simulink model "exercise2_1"  (R2025a)
settings: Solver=FixedStepAuto  StartTime=0.0  StopTime=20  FixedStep=1e-5  RelTol=1e-3
values from neighbouring files (symbols this model uses):
  B = 0    [exercise2_1.m]
  J = 2.52e-3    (= 0.00252)    [exercise2_1.m]
  K = 0.4078    [exercise2_1.m]
  Ki = 0.8    [exercise2_1.m]
  Kp = 0.1    [exercise2_1.m]
  L = 1.7e-3    (= 0.0017)    [exercise2_1.m]
  R = 0.26    [exercise2_1.m]
  wn = 2*pi*350    (= 2199.11485751)    [exercise2_1.m]
  Ww = 60    [exercise2_1.m]
  zeta = 0.707    [exercise2_1.m]
libraries: simulink_extras x1, simulink x1
settings Model: Creator=moon  LastModifiedBy=New

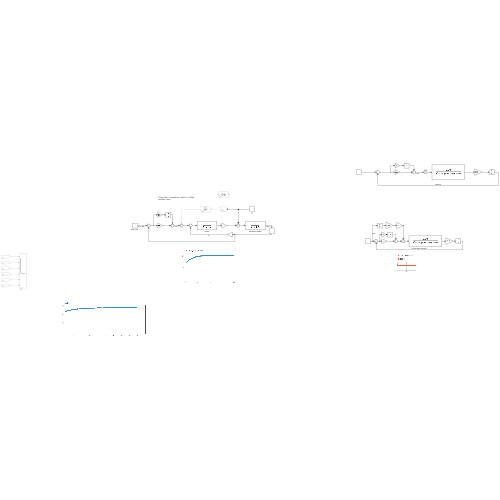
[thumbnail: Simulink's stored preview of the top-level diagram]
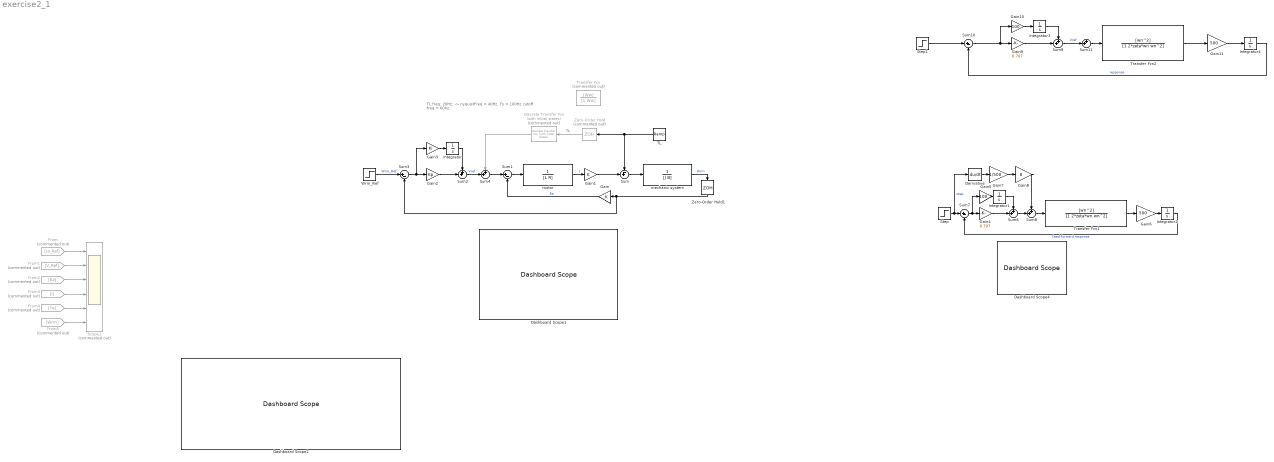
== system exercise2_1 ==
  note: TL freq: 20Hz; -> nyquistFreq = 40Hz, Fs = 100Hz
      | cutoff freq = 60hz.
  Dashboard Scope1 : DashboardScope  FontColor=[0.0, 0.0, 0.0]
  Dashboard Scope2 : DashboardScope  UpdateMode=Scroll  FontColor=[0.0, 0.0, 0.0]
  Dashboard Scope4 : DashboardScope  FontColor=[0.0, 0.0, 0.0]
  Derivative : Derivative
  Discrete Transfer Fcn (with initial states) : simulink_extras/Additional Discrete/Discrete Transfer Fcn (with initial states)  Commented=on  N=[3 3]  D=[6 3]  X0=[0]  TS=.1
  From : From  Commented=on  GotoTag=Ia_Ref
  From1 : From  Commented=on  GotoTag=V_Ref
  From2 : From  Commented=on  GotoTag=Ea
  From3 : From  Commented=on  GotoTag=I
  From4 : From  Commented=on  GotoTag=Te
  From5 : From  Commented=on  GotoTag=Wrm
  Gain : Gain  Gain=K
  Gain1 : Gain  Gain=K
  Gain10 : Gain  Gain=100
  Gain11 : Gain  Gain=500
  Gain2 : Gain  Gain=Kp
  Gain3 : Gain  Gain=Ki
  Gain4 : Gain  Gain=0.707
  Gain5 : Gain  Gain=100
  Gain6 : Gain  Gain=500
  Gain7 : Gain  Gain=1/500
  Gain8 : Gain  Gain=8
  Gain9 : Gain  Gain=0.707
  Integrator{,1..4} (5 alike) : Integrator
  Scope1 : Scope  Commented=on  NumInputPorts=6
      settings: ActiveDisplayYMinimum=-17.5  ActiveDisplayYMaximum=157.5
  Step : Step  Time=0.02  SampleTime=0
  Step1 : Step  Time=0.02  SampleTime=0
  Sum : Sum  Inputs=-+|
  Sum{1,3,7,10} (4 alike) : Sum  Inputs=|+-
  Sum{2,4,6,8..9,11} (6 alike) : Sum  Inputs=++|
  TL : simulink/Sources/Ramp  slope=100  start=0  InitialOutput=0
  Transfer Fcn : TransferFcn  Commented=on  Numerator=[Ww]  Denominator=[1 Ww]
  Transfer Fcn1 : TransferFcn  Numerator=[wn^2]  Denominator=[1 2*zeta*wn wn^2]
  Transfer Fcn2 : TransferFcn  Numerator=[wn^2]  Denominator=[1 2*zeta*wn wn^2]
  Wrm_Ref : Step  Time=0.1  After=200  SampleTime=0
  Zero-Order Hold : ZeroOrderHold  Commented=on  SampleTime=0.05
  Zero-Order Hold1 : ZeroOrderHold  SampleTime=1e-4
  mechanic system : TransferFcn  Denominator=[J B]
  motor : TransferFcn  Denominator=[L R]
  wires:
  motor/1 -> Gain1/1  "I"
  Gain1/1 -> Sum/2
  Sum/1 -> mechanic system/1
  Gain/1 -> Sum1/2  "Ea"
  Sum1/1 -> motor/1
  Gain3/1 -> Integrator/1
  Integrator/1 -> Sum2/1
  Gain2/1 -> Sum2/2
  Sum3/1 -> Gain3/1, Gain2/1
  Sum2/1 -> Sum4/2  "Vref"
  From/1 -> Scope1/1
  From2/1 -> Scope1/3
  From3/1 -> Scope1/4
  From4/1 -> Scope1/5
  From5/1 -> Scope1/6
  From1/1 -> Scope1/2
  Wrm_Ref/1 -> Sum3/1  "Wrm_Ref"
  TL/1 -> Zero-Order Hold/1, Sum/1
  Zero-Order Hold/1 -> Discrete Transfer Fcn (with initial states)/1  "TL"
  Zero-Order Hold1/1 -> Gain/1, Sum3/2
  mechanic system/1 -> Zero-Order Hold1/1  "Wrm"
  Sum4/1 -> Sum1/1
  Integrator1/1 -> Sum6/1
  Gain4/1 -> Sum6/2
  Gain5/1 -> Integrator1/1
  Step/1 -> Derivative/1, Sum7/1  "step"
  Sum7/1 -> Gain5/1, Gain4/1
  Gain6/1 -> Integrator2/1
  Transfer Fcn1/1 -> Gain6/1
  Sum6/1 -> Sum8/2
  Integrator2/1 -> Sum7/2  "feed-forward response"
  Derivative/1 -> Gain7/1
  Gain7/1 -> Gain8/1
  Sum8/1 -> Transfer Fcn1/1
  Gain8/1 -> Sum8/1
  Sum10/1 -> Gain10/1, Gain9/1
  Gain11/1 -> Integrator4/1
  Integrator3/1 -> Sum9/1
  Gain10/1 -> Integrator3/1
  Gain9/1 -> Sum9/2
  Sum9/1 -> Sum11/2  "Vref"
  Sum11/1 -> Transfer Fcn2/1
  Transfer Fcn2/1 -> Gain11/1
  Integrator4/1 -> Sum10/2  "response"
  Step1/1 -> Sum10/1
  Discrete Transfer Fcn (with initial states)/1 -> Sum4/1
